simulink model "ExampleAtmosphere"  (R2024a)
settings: Solver=FixedStepAuto  StartTime=0.0  StopTime=inf  FixedStep=0.02  RelTol=1e-3  EnableMultiTasking=on
undefined symbols (not defined in the file): atmosphericScattering, basicProperties, position, quaternion, sunDisc
libraries: PRISMA x7, simulink_extras x1, GenericTarget x1
settings Model: Creator=damerius  LastModifiedBy=Scythe
settings SolverCC: ConcurrentTasks=on  AlgebraicLoopSolver=TrustRegion  PositivePriorityOrder=on
settings DataIOCC: SaveOutput=off  SignalLogging=off  DSMLogging=off  SaveTime=off  ReturnWorkspaceOutputs=off
settings OptimizationCC: DefaultParameterBehavior=Inlined  ReuseModelBlockBuffer=off  ZeroExternalMemoryAtStartup=off  ZeroInternalMemoryAtStartup=off  SimCompilerOptimization=on
settings DebuggingCC: UnconnectedInputMsg=warning  UnconnectedOutputMsg=warning  UnconnectedLineMsg=warning
settings HardwareCC: ProdBitPerLong=64  ProdHWDeviceType=Intel->x86-64 (Linux 64)
settings ModelReferenceCC: EnableRefExpFcnMdlSchedulingChecks=on
settings SFSimCC: SimParseCustomCode=off  SimGenImportedTypeDefs=on  SimTargetLang=C++
settings RTWCC: GenCodeOnly=on  PackageGeneratedCodeAndArtifacts=on  PackageName=PackNGo  RTWVerbose=off  BuildConfiguration=Faster Runs  TargetLang=C++  GPUComputeCapability=3.5  DLArmComputeVersion=19.05
settings CodeAppCC: ForceParamTrailComments=on  MaxIdLength=95  MATLABSourceComments=on  UseSimReservedNames=on
settings GRTTargetCC: TargetLangStandard=C++11 (ISO)  GenerateFullHeader=off  MatFileLogging=off  CodeInterfacePackaging=C++ class

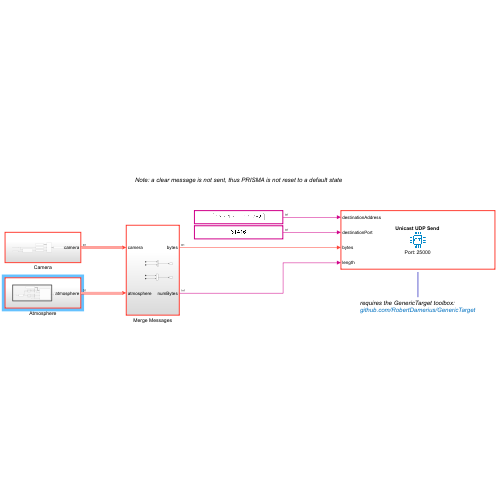
[thumbnail: Simulink's stored preview of the top-level diagram]
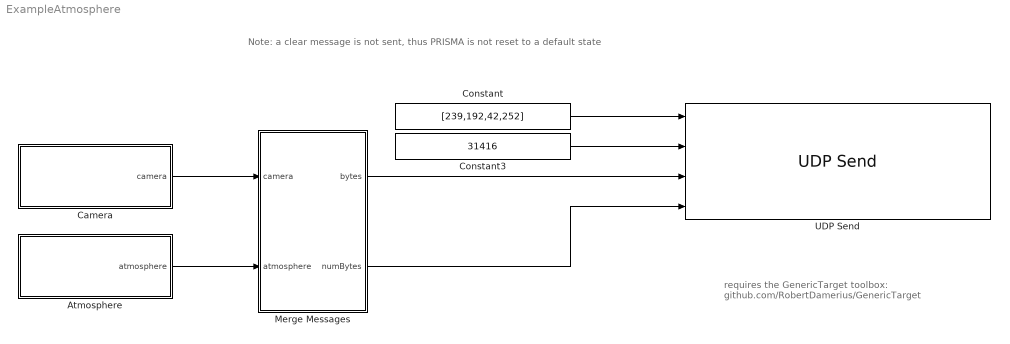
== system ExampleAtmosphere ==
  note: Note: a clear message is not sent, thus PRISMA is not reset to a default state
  note: requires the GenericTarget toolbox:
      | github.com/RobertDamerius/GenericTarget
  Atmosphere : Subsystem
  Camera : Subsystem
  Constant : Constant  Value=[239,192,42,252]  OutDataTypeStr=uint8
  Constant3 : Constant  Value=31416  OutDataTypeStr=uint16
  Merge Messages : Subsystem
  UDP Send : GenericTarget/Interface/UDP Send  showDetails=off  interfacePort=25000  interfaceIP=[0,0,0,0]  deviceName=''  prioritySocket=6  allowBroadcast=off  SampleTime=-1
      settings: SourceProductName=Generic Target
  wires:
  Constant/1 -> UDP Send/1
  Constant3/1 -> UDP Send/2
  Camera/1(camera) -> Merge Messages/1(camera)
  Merge Messages/1(bytes) -> UDP Send/3
  Merge Messages/2(numBytes) -> UDP Send/4
  Atmosphere/1(atmosphere) -> Merge Messages/2(atmosphere)

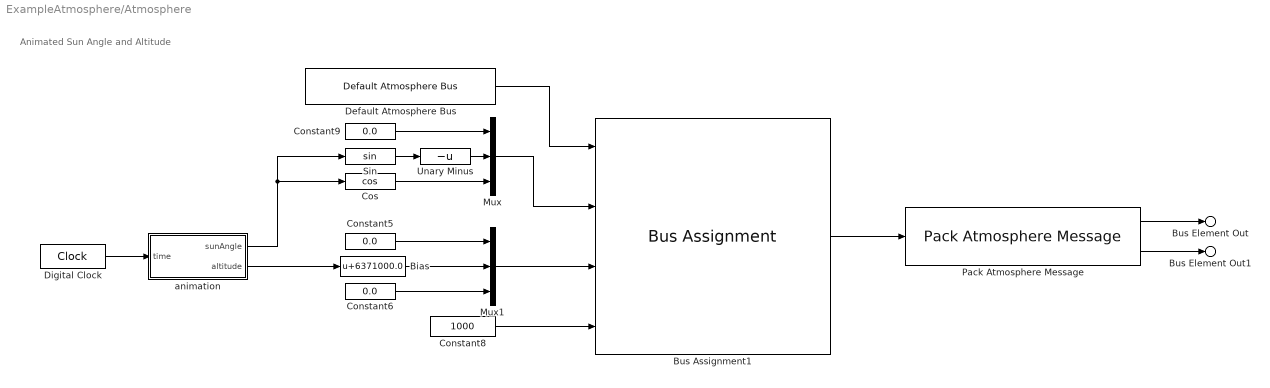
== system ExampleAtmosphere/Atmosphere ==
  note: Animated Sun Angle and Altitude
  Bias : Bias  Bias=6371000.0  SaturateOnIntegerOverflow=off
  Bus Assignment1 : BusAssignment  AssignedSignals=basicProperties.sunLightDirection,atmosphericScattering.eyePosition,sunDisc.intensity
  Constant5 : Constant  Value=0.0
  Constant6 : Constant  Value=0.0
  Constant8 : Constant  Value=1000
  Constant9 : Constant  Value=0.0
  Cos : Trigonometry  Operator=cos
  Default Atmosphere Bus : PRISMA/Default Atmosphere Bus
      settings: SourceProductName=PRISMA
  Digital Clock : DigitalClock  SampleTime=0.02
  Mux : Mux  Inputs=3
  Mux1 : Mux  Inputs=3
  Pack Atmosphere Message : PRISMA/Pack Atmosphere Message
      settings: SourceProductName=PRISMA
  Sin : Trigonometry
  Unary Minus : UnaryMinus
  animation : Subsystem
  Bus Element Out : Outport  PortName=atmosphere  Element=bytes
  Bus Element Out1 : Outport  PortName=atmosphere  Element=numBytes
  wires:
  Pack Atmosphere Message/2 -> Bus Element Out1/1
  Pack Atmosphere Message/1 -> Bus Element Out/1
  Constant8/1 -> Bus Assignment1/4
  animation/2(altitude) -> Bias/1
  Bias/1 -> Mux1/2
  Constant6/1 -> Mux1/3
  Constant5/1 -> Mux1/1
  Mux1/1 -> Bus Assignment1/3
  Mux/1 -> Bus Assignment1/2
  Default Atmosphere Bus/1 -> Bus Assignment1/1
  animation/1(sunAngle) -> Sin/1, Cos/1
  Unary Minus/1 -> Mux/2
  Constant9/1 -> Mux/1
  Sin/1 -> Unary Minus/1
  Cos/1 -> Mux/3
  Digital Clock/1 -> animation/1(time)
  Bus Assignment1/1 -> Pack Atmosphere Message/1

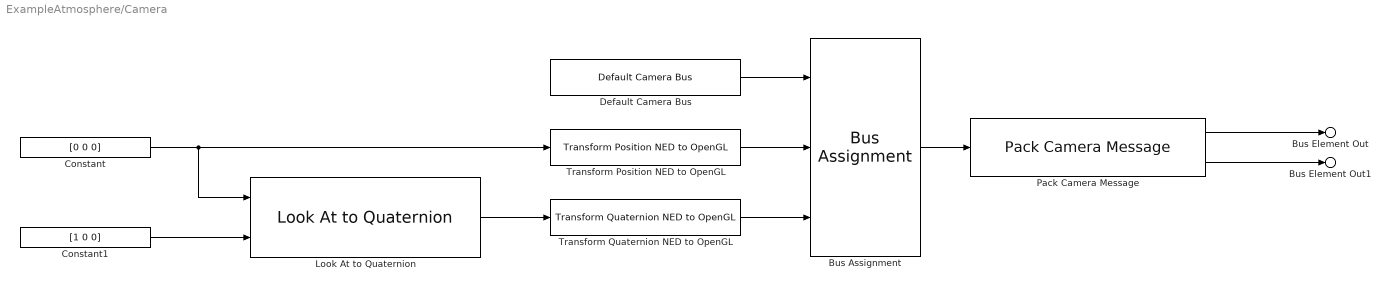
== system ExampleAtmosphere/Camera ==
  Bus Assignment : BusAssignment  AssignedSignals=position,quaternion
  Constant : Constant  Value=[0 0 0]
  Constant1 : Constant  Value=[1 0 0]
  Default Camera Bus : PRISMA/Default Camera Bus
      settings: SourceProductName=PRISMA
  Look At to Quaternion : PRISMA/Transformation/Look At to Quaternion
      settings: SourceProductName=PRISMA
  Pack Camera Message : PRISMA/Pack Camera Message
      settings: SourceProductName=PRISMA
  Transform Position NED to OpenGL : PRISMA/Transformation/Transform Position NED to OpenGL
      settings: SourceProductName=PRISMA
  Transform Quaternion NED to OpenGL : PRISMA/Transformation/Transform Quaternion NED to OpenGL
      settings: SourceProductName=PRISMA
  Bus Element Out : Outport  PortName=camera  Element=bytes
  Bus Element Out1 : Outport  PortName=camera  Element=numBytes
  wires:
  Default Camera Bus/1 -> Bus Assignment/1
  Bus Assignment/1 -> Pack Camera Message/1
  Transform Position NED to OpenGL/1 -> Bus Assignment/2
  Transform Quaternion NED to OpenGL/1 -> Bus Assignment/3
  Look At to Quaternion/1 -> Transform Quaternion NED to OpenGL/1
  Constant/1 -> Look At to Quaternion/1, Transform Position NED to OpenGL/1
  Constant1/1 -> Look At to Quaternion/2
  Pack Camera Message/1 -> Bus Element Out/1
  Pack Camera Message/2 -> Bus Element Out1/1

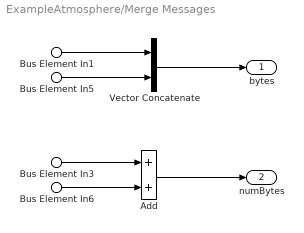
== system ExampleAtmosphere/Merge Messages ==
  Bus Element In1 : Inport  PortName=camera  Element=bytes
  Bus Element In3 : Inport  PortName=camera  Element=numBytes
  Bus Element In5 : Inport  Port=2  PortName=atmosphere  Element=bytes
  Bus Element In6 : Inport  Port=2  PortName=atmosphere  Element=numBytes
  Add : Sum
  Vector Concatenate : Concatenate
  bytes : Outport
  numBytes : Outport  Port=2
  wires:
  Bus Element In1/1 -> Vector Concatenate/1
  Bus Element In3/1 -> Add/1
  Vector Concatenate/1 -> bytes/1
  Add/1 -> numBytes/1
  Bus Element In5/1 -> Vector Concatenate/2
  Bus Element In6/1 -> Add/2

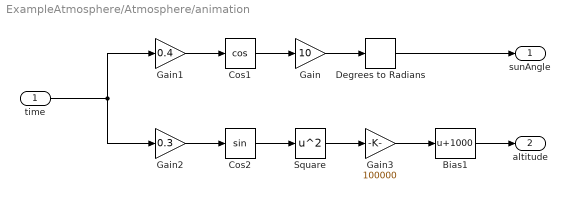
== system ExampleAtmosphere/Atmosphere/animation ==
  time : Inport
  Bias1 : Bias  Bias=1000  SaturateOnIntegerOverflow=off
  Cos1 : Trigonometry  Operator=cos
  Cos2 : Trigonometry
  Degrees to Radians : simulink_extras/Transformations/Degrees to Radians
  Gain : Gain  Gain=10
  Gain1 : Gain  Gain=0.4
  Gain2 : Gain  Gain=0.3
  Gain3 : Gain  Gain=100000
  Square : Math  Operator=square
  sunAngle : Outport
  altitude : Outport  Port=2
  wires:
  time/1 -> Gain2/1, Gain1/1
  Square/1 -> Gain3/1
  Degrees to Radians/1 -> sunAngle/1
  Bias1/1 -> altitude/1
  Gain/1 -> Degrees to Radians/1
  Gain2/1 -> Cos2/1
  Gain3/1 -> Bias1/1
  Gain1/1 -> Cos1/1
  Cos1/1 -> Gain/1
  Cos2/1 -> Square/1
